simulink model "Dynamic_obstacle_avoidance_PIL"  (R2019a)
settings: Solver=VariableStepAuto  StartTime=0.0  StopTime=distance/V  MaxStep=1e-3  RelTol=1e-3  EnableMultiTasking=on
undefined symbols (not defined in the file): extended_map, fakeObs, Lw, obstacle, p, param, Ts, u0, WMV, WMVR, WOV, x0_dyn
libraries: simulink x4, mpclib x2
settings Model: Creator=The MathWorks, Inc.  LastModifiedBy=djtn
settings SolverCC: AlgebraicLoopSolver=LineSearch  MinimalZcImpactIntegration=on
settings DataIOCC: LimitDataPoints=on  SaveFormat=Array  SaveOutput=off  DSMLogging=off  SaveTime=off  ReturnWorkspaceOutputs=off
settings OptimizationCC: DefaultParameterBehavior=Inlined  UseDivisionForNetSlopeComputation=on  EnhancedBackFolding=on  PassReuseOutputArgsAs=Individual arguments  OptimizeBlockOrder=speed  DifferentSizesBufferReuse=on  OptimizationCustomize=off
settings DebuggingCC: AlgebraicLoopMsg=none  UnderspecifiedInitializationDetection=Classic  MergeDetectMultiDrivingBlocksExec=none  SolverPrmCheckMsg=warning  ParameterTunabilityLossMsg=error  AllowSymbolicDim=off  StateNameClashWarn=warning  SFUnexpectedBacktrackingDiag=warning  SFNoUnconditionalDefaultTransitionDiag=warning  SFExecutionAtInitializationDiag=none  UnderSpecifiedDimensionMsg=warning  ArithmeticOperatorsInVariantConditions=warning
settings HardwareCC: ProdBitPerPointer=32  ProdBitPerSizeT=32  ProdBitPerPtrDiffT=32  ProdLargestAtomicInteger=Long  ProdWordSize=32  ProdHWDeviceType=STM32CortexM
settings ModelReferenceCC: PropagateSignalLabelsOutOfModel=off
settings SFSimCC: SimUseLocalCustomCode=off  MATLABDynamicMemAlloc=off
settings RTWCC: SystemTargetFile=stm32.tlc  TemplateMakefile=stm32.tmf  Description=stm32 (Embedded Target)  GenerateReport=on  RTWUseLocalCustomCode=off  IncludeHyperlinkInReport=on  GenerateTraceInfo=on  GenerateTraceReport=on  GenerateTraceReportSl=on  GenerateTraceReportSf=on  GenerateTraceReportEml=on  CheckMdlBeforeBuild=Warning
settings CodeAppCC: ForceParamTrailComments=on  IgnoreCustomStorageClasses=off  MaxIdLength=64  OperatorAnnotations=on  SimulinkDataObjDesc=on  SFDataObjDesc=on  CustomSymbolStrType=$N$R$M  SimulinkBlockComments=off
settings STFCustomTargetCC: CodeReplacementLibrary=ARM CMSIS SIN COS  MultiwordLength=256  ParMdlRefBuildCompliant=on  IncludeMdlTerminateFcn=off  CombineOutputUpdateFcns=on  ERTCustomFileBanners=on  SupportContinuousTime=off  SupportNonInlinedSFcns=off  RemoveResetFunc=on  MATLABClassNameForMDSCustomization=Simulink.SoftwareTarget.ERTCustomization  GRTInterface=off  SystemTargetFile=stm32.tlc
settings ERTTargetCC: CodeReplacementLibrary=ARM CMSIS SIN COS  CompOptLevelCompliant=off  ConcurrentExecutionCompliant=off  IncludeMdlTerminateFcn=off  ModelStepFunctionPrototypeControlCompliant=off  CPPClassGenCompliant=off  UseToolchainInfoCompliant=off  ExtModeStaticAllocSize=256  ExtModeMexFile=ext_serial_win32_comm  ExtModeMexArgs=0,1,115200,10  InlinedParameterPlacement=NonHierarchical  ERTSrcFileBannerTemplate=sourceFileTemplate.cgt  ERTHdrFileBannerTemplate=sourceFileTemplate.cgt  ERTDataSrcFileTemplate=sourceFileTemplate.cgt  ERTDataHdrFileTemplate=sourceFileTemplate.cgt  ERTCustomFileTemplate=customRoutineProcess.tlc
settings ConfigComp: CovMetricSettings=dw  CovSaveCumulativeToWorkspaceVar=on  CovSaveSingleToWorkspaceVar=on  CovExternalEMLEnable=off  CovSFcnEnable=off
settings SimscapeCC: SimscapeNormalizeSystem=off  SimscapeNominalValues="[{\"value\":\"10\",\"unit\":\"V\"},{\"value\":\"1\",\"unit\":\"A\"},{\"value\":\"10\",\"unit\":\"N*m\"},{\"value\":\"10\",\"unit\":\"bar\"},{\"value\":\"100\",\"unit\":\"kJ/kg\"},{\"value\":\"1\",\"unit\":\"kW\"},{\"value\":\"300\",\"unit\":\"K\"},{\"value\":\"100\",\"unit\":\"cm^3/s\"},{\"value\":\"1\",\"unit\":\"kN\"},{\"value\":\"1\",\"unit\":\"g/cm^3\"},{\"value\":\"1\",\"unit\":\"l\"},{\"value\":\"1\",\"unit\":\"cm^2\"},{\"value\":\"60\",\"unit\":\"Hz\"}]"
settings ConfigurationSet: Description=SimMechanics 2G
settings ExplorerConfigSet: InternalSimMechanicsExplorerSettings="<ExplorerConfiguration><canonicalview>default</canonicalview><AnimationSetting><BasePlaybackSpeed>1.0</BasePlaybackSpeed><PlaybackSpeedFactor>1.0</PlaybackSpeedFactor></AnimationSetting><TilePanel><TileInfo><Tiles Columns=\"1\" Count=\"1\" Rows=\"1\"><Column Left=\"2\" Weight=\"1\"/><Column Left=\"1552\"/><Row Top=\"2\" Weight=\"1\"/><Row Top=\"932\"/><Tile Height=\"1\" Width=\"1\" X=\"0\" Y=\"0\"/></Tiles></TileInfo><SceneInfo><SceneViewer><BGColor><R>0.60000002384185791</R><G>0.60000002384185791</G><B>0.60000002384185791</B></BGColor><Camera><Position><X>0.027865189060748197</X><Y>-2.5719092456962986</Y><Z>0.23157896538506753</Z></Position><Center><X>0.62659712312732463</X><Y>-0.46110119691712204</Y><Z>0.22087365386473376</Z></Center><Up><X>-0.0079438354874226333</X><Y>0.0073246425924307582</Y><Z>0.99994162084025784</Z></Up><Left>-0.24533778208815546</Left><Right>0.24533778208815546</Right><Bottom>-0.79734779727023208</Bottom><Top>0.79734779727023208</Top></Camera></SceneViewer></SceneInfo></TilePanel></ExplorerConfiguration>"

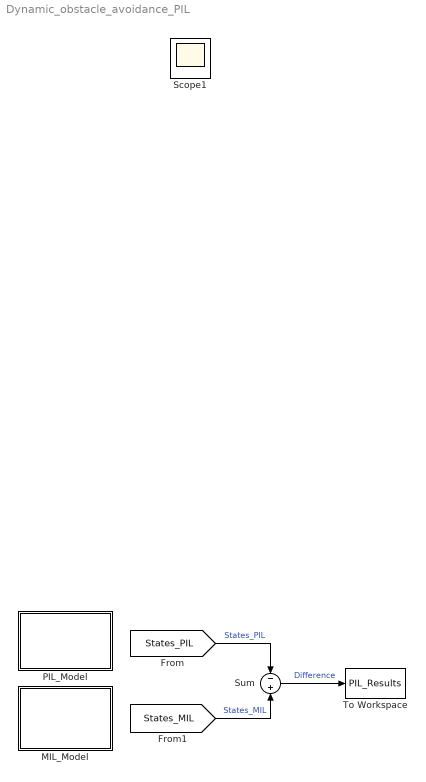
== system Dynamic_obstacle_avoidance_PIL ==
  MIL_Model : Subsystem
  PIL_Model : Subsystem
  Sum : Sum  Inputs=-+
  To Workspace : ToWorkspace  VariableName=PIL_Results  SampleTime=Ts
  Scope1 : Scope
  wires:
  [States_PIL] -> Sum/1  "States_PIL"
  [States_MIL] -> Sum/2  "States_MIL"
  Sum/1 -> To Workspace/1  "Difference"

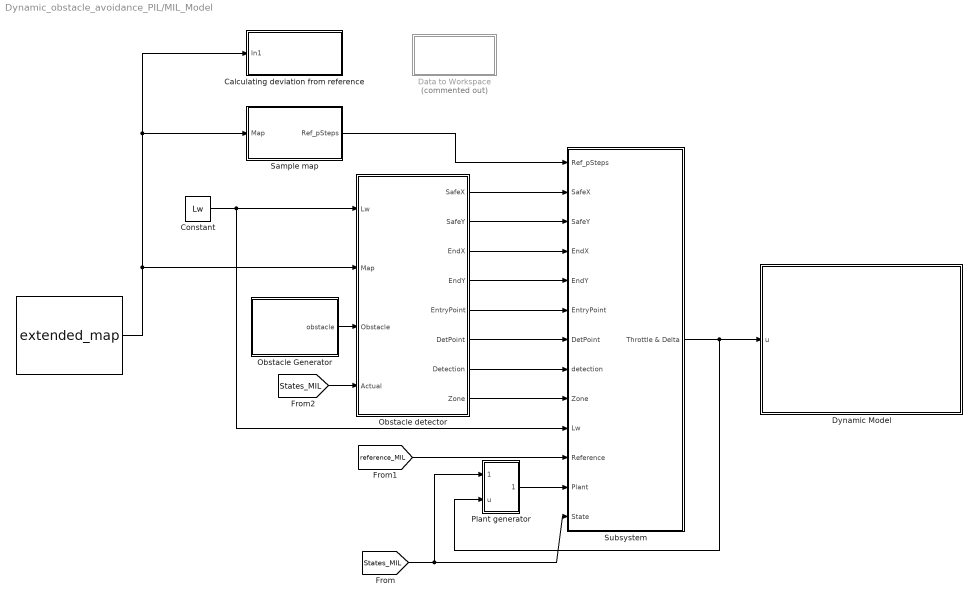
== system Dynamic_obstacle_avoidance_PIL/MIL_Model ==
  "  " : Constant  Value=extended_map  SampleTime=Ts
      mask Display: image('creative_map_city.jpg')
  Calculating deviation from reference : Subsystem
  Constant : Constant  Value=Lw
  Data to Workspace : Subsystem  Commented=on
  Dynamic Model : Subsystem
      mask Display: image('hyundai_verna.jpg')
  Obstacle Generator : Subsystem
  Obstacle detector : Subsystem
  Plant generator : Subsystem
  Sample map : Subsystem
  Subsystem : Subsystem
  wires:
  Obstacle detector/8(Zone) -> Subsystem/9(Zone)
  Obstacle detector/7(Detection) -> Subsystem/8(detection)
  Obstacle detector/6(DetPoint) -> Subsystem/7(DetPoint)
  Obstacle detector/5(EntryPoint) -> Subsystem/6(EntryPoint)
  Obstacle detector/4(EndY) -> Subsystem/5(EndY)
  Obstacle detector/3(EndX) -> Subsystem/4(EndX)
  Obstacle detector/2(SafeY) -> Subsystem/3(SafeY)
  Obstacle detector/1(SafeX) -> Subsystem/2(SafeX)
  [States_MIL] -> Obstacle detector/4(Actual)
  Obstacle Generator/1(obstacle) -> Obstacle detector/3(Obstacle)
  Sample map/1(Ref_pSteps) -> Subsystem/1(Ref_pSteps)
  "  "/1 -> Obstacle detector/2(Map), Sample map/1(Map), Calculating deviation from reference/1(In1)
  Plant generator/1(Out1) -> Subsystem/12(Plant)
  [reference_MIL] -> Subsystem/11(Reference)
  Subsystem/1(Throttle & Delta) -> Plant generator/2(u), Dynamic Model/1(u)
  Constant/1 -> Subsystem/10("Lw "), Obstacle detector/1(Lw)
  [States_MIL] -> Subsystem/13(State), Plant generator/1(State)

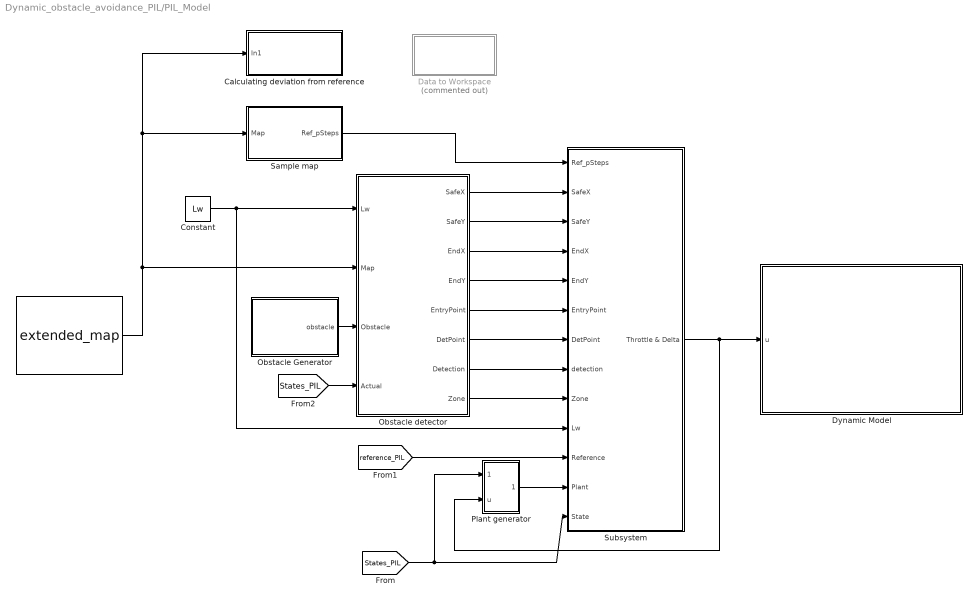
== system Dynamic_obstacle_avoidance_PIL/PIL_Model ==
  "  " : Constant  Value=extended_map  SampleTime=Ts
      mask Display: image('creative_map_city.jpg')
  Calculating deviation from reference : Subsystem
  Constant : Constant  Value=Lw
  Data to Workspace : Subsystem  Commented=on
  Dynamic Model : Subsystem
      mask Display: image('hyundai_verna.jpg')
  Obstacle Generator : Subsystem
  Obstacle detector : Subsystem
  Plant generator : Subsystem
  Sample map : Subsystem
  Subsystem : Subsystem
  wires:
  [States_PIL] -> Plant generator/1(State), Subsystem/13(State)
  Constant/1 -> Obstacle detector/1(Lw), Subsystem/10("Lw ")
  Subsystem/1(Throttle & Delta) -> Dynamic Model/1(u), Plant generator/2(u)
  [reference_PIL] -> Subsystem/11(Reference)
  Plant generator/1(Out1) -> Subsystem/12(Plant)
  "  "/1 -> Calculating deviation from reference/1(In1), Sample map/1(Map), Obstacle detector/2(Map)
  Sample map/1(Ref_pSteps) -> Subsystem/1(Ref_pSteps)
  Obstacle Generator/1(obstacle) -> Obstacle detector/3(Obstacle)
  [States_PIL] -> Obstacle detector/4(Actual)
  Obstacle detector/1(SafeX) -> Subsystem/2(SafeX)
  Obstacle detector/2(SafeY) -> Subsystem/3(SafeY)
  Obstacle detector/3(EndX) -> Subsystem/4(EndX)
  Obstacle detector/4(EndY) -> Subsystem/5(EndY)
  Obstacle detector/5(EntryPoint) -> Subsystem/6(EntryPoint)
  Obstacle detector/6(DetPoint) -> Subsystem/7(DetPoint)
  Obstacle detector/7(Detection) -> Subsystem/8(detection)
  Obstacle detector/8(Zone) -> Subsystem/9(Zone)

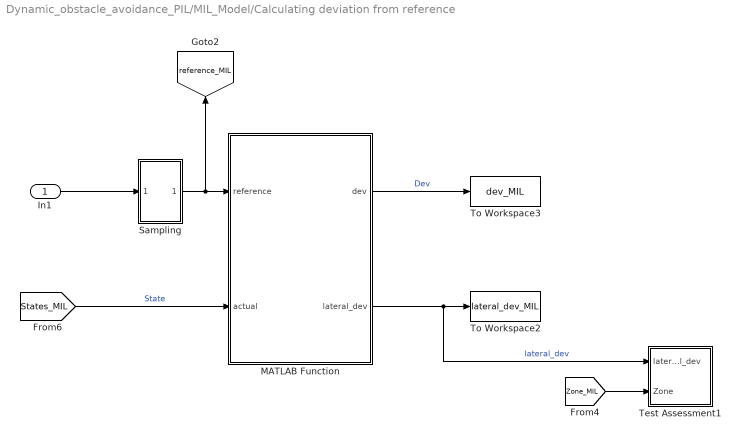
== system Dynamic_obstacle_avoidance_PIL/MIL_Model/Calculating deviation from reference ==
  In1 : Inport
  MATLAB Function : MATLAB Function  TreatAsAtomicUnit=on
  Sampling : Subsystem
  Test Assessment1 : Test Sequence  TreatAsAtomicUnit=on
  To Workspace2 : ToWorkspace  VariableName=lateral_dev_MIL  SampleTime=Ts
  To Workspace3 : ToWorkspace  VariableName=dev_MIL  SampleTime=-1
  tag scope: reference_MIL=global
  wires:
  [Zone_MIL] -> Test Assessment1/2(Zone)
  MATLAB Function/2(lateral_dev) -> Test Assessment1/1(lateral_dev), To Workspace2/1  "lateral_dev"
  MATLAB Function/1(dev) -> To Workspace3/1  "Dev"
  In1/1 -> Sampling/1(In1)
  Sampling/1(Out1) -> [reference_MIL], MATLAB Function/1(reference)
  [States_MIL] -> MATLAB Function/2(actual)  "State"

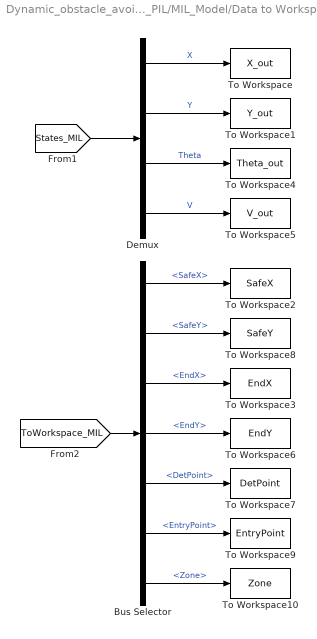
== system Dynamic_obstacle_avoidance_PIL/MIL_Model/Data to Workspace ==
  Bus Selector : BusSelector  OutputSignals=SafeX,SafeY,EndX,EndY,DetPoint,EntryPoint,Zone
  Demux : Demux
  To Workspace : ToWorkspace  VariableName=X_out  SampleTime=Ts
  To Workspace1 : ToWorkspace  VariableName=Y_out  SampleTime=Ts
  To Workspace10 : ToWorkspace  VariableName=Zone  SampleTime=-1
  To Workspace2 : ToWorkspace  VariableName=SafeX  SampleTime=-1
  To Workspace3 : ToWorkspace  VariableName=EndX  SampleTime=-1
  To Workspace4 : ToWorkspace  VariableName=Theta_out  SampleTime=Ts
  To Workspace5 : ToWorkspace  VariableName=V_out  SampleTime=Ts
  To Workspace6 : ToWorkspace  VariableName=EndY  SampleTime=-1
  To Workspace7 : ToWorkspace  VariableName=DetPoint  SampleTime=-1
  To Workspace8 : ToWorkspace  VariableName=SafeY  SampleTime=-1
  To Workspace9 : ToWorkspace  VariableName=EntryPoint  SampleTime=-1
  wires:
  Bus Selector/7 -> To Workspace10/1  "<Zone>"
  Bus Selector/6 -> To Workspace9/1  "<EntryPoint>"
  Bus Selector/5 -> To Workspace7/1  "<DetPoint>"
  Bus Selector/4 -> To Workspace6/1  "<EndY>"
  Bus Selector/3 -> To Workspace3/1  "<EndX>"
  Bus Selector/2 -> To Workspace8/1  "<SafeY>"
  Bus Selector/1 -> To Workspace2/1  "<SafeX>"
  [ToWorkspace_MIL] -> Bus Selector/1
  Demux/1 -> To Workspace/1  "X"
  [States_MIL] -> Demux/1
  Demux/4 -> To Workspace5/1  "V"
  Demux/2 -> To Workspace1/1  "Y"
  Demux/3 -> To Workspace4/1  "Theta"

== system Dynamic_obstacle_avoidance_PIL/MIL_Model/Dynamic Model ==
  u : Inport
  Bus Creator1 : BusCreator  Inputs=4
  C_r : Constant  Value=param  SampleTime=Ts
  Dynamic_Model : MATLAB Function  TreatAsAtomicUnit=on
  Integrator : Integrator  InitialCondition=x0_dyn
  Lateral Acceleration Assessment : Test Sequence  TreatAsAtomicUnit=on
  Selector2 : Selector  InputPortWidth=6  IndexOptions=Index vector (dialog)  Indices=[5]  OutputSizes=1
  tag scope: States_MIL=global
  wires:
  u/1 -> Dynamic_Model/2(u)
  C_r/1 -> Dynamic_Model/3(param)
  Integrator/1 -> Dynamic_Model/1(x)
  Dynamic_Model/5(v) -> Bus Creator1/4  "V"
  Dynamic_Model/2(X) -> Bus Creator1/1  "X"
  Dynamic_Model/4(yaw) -> Bus Creator1/3  "yaw"
  Dynamic_Model/1(xdot) -> Selector2/1, Integrator/1
  Selector2/1 -> Lateral Acceleration Assessment/1(Lateral_acceleration)  "Lateral acceleration"
  Bus Creator1/1 -> [States_MIL]
  Dynamic_Model/3(Y) -> Bus Creator1/2  "Y"

== system Dynamic_obstacle_avoidance_PIL/MIL_Model/Obstacle Generator ==
  Constant4 : Constant  Value=obstacle
  FakeObs : Constant  Value=fakeObs
  From Workspace : FromWorkspace  VariableName=extended_obs  SampleTime=0
  From Workspace1 : FromWorkspace  VariableName=extended_obs2  SampleTime=0
  Matrix Concatenate : Concatenate  NumInputs=4  Mode=Multidimensional array
  Transpose : Math  Operator=transpose  SaturateOnIntegerOverflow=on
  Transpose1 : Math  Operator=transpose  SaturateOnIntegerOverflow=on
  obstacle : Outport
  wires:
  FakeObs/1 -> Matrix Concatenate/4
  Transpose1/1 -> Matrix Concatenate/3
  From Workspace1/1 -> Transpose1/1
  Transpose/1 -> Matrix Concatenate/2
  Constant4/1 -> Matrix Concatenate/1
  Matrix Concatenate/1 -> obstacle/1
  From Workspace/1 -> Transpose/1

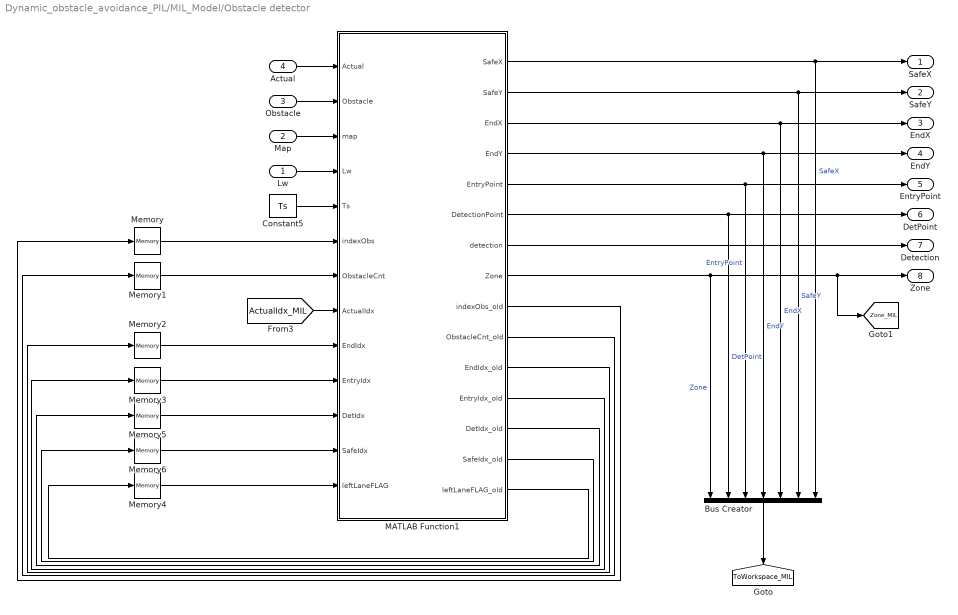
== system Dynamic_obstacle_avoidance_PIL/MIL_Model/Obstacle detector ==
  Lw : Inport
  Map : Inport  Port=2
  Obstacle : Inport  Port=3
  Actual : Inport  Port=4
  Bus Creator : BusCreator  Inputs=7
  Constant5 : Constant  Value=Ts
  MATLAB Function1 : MATLAB Function  TreatAsAtomicUnit=on
  Memory{,1..6} (7 alike) : Memory
  SafeX : Outport
  SafeY : Outport  Port=2
  EndX : Outport  Port=3
  EndY : Outport  Port=4
  EntryPoint : Outport  Port=5
  DetPoint : Outport  Port=6
  Detection : Outport  Port=7
  Zone : Outport  Port=8
  tag scope: ToWorkspace_MIL=global, Zone_MIL=global
  wires:
  Map/1 -> MATLAB Function1/3(map)
  MATLAB Function1/12(EntryIdx_old) -> Memory3/1
  MATLAB Function1/13(DetIdx_old) -> Memory5/1
  MATLAB Function1/14(SafeIdx_old) -> Memory6/1
  Constant5/1 -> MATLAB Function1/5(Ts)
  Memory/1 -> MATLAB Function1/6(indexObs)
  MATLAB Function1/9(indexObs_old) -> Memory/1
  MATLAB Function1/4(EndY) -> Bus Creator/4, EndY/1  "EndY"
  MATLAB Function1/3(EndX) -> Bus Creator/5, EndX/1  "EndX"
  Obstacle/1 -> MATLAB Function1/2(Obstacle)
  Memory5/1 -> MATLAB Function1/11(DetIdx)
  MATLAB Function1/7(detection) -> Detection/1
  Memory2/1 -> MATLAB Function1/9(EndIdx)
  Memory6/1 -> MATLAB Function1/12(SafeIdx)
  Memory4/1 -> MATLAB Function1/13(leftLaneFLAG)
  Memory1/1 -> MATLAB Function1/7(ObstacleCnt)
  MATLAB Function1/5(EntryPoint) -> EntryPoint/1, Bus Creator/3  "EntryPoint"
  Bus Creator/1 -> [ToWorkspace_MIL]
  MATLAB Function1/2(SafeY) -> Bus Creator/6, SafeY/1  "SafeY"
  Actual/1 -> MATLAB Function1/1(Actual)
  MATLAB Function1/1(SafeX) -> Bus Creator/7, SafeX/1  "SafeX"
  MATLAB Function1/15(leftLaneFLAG_old) -> Memory4/1
  MATLAB Function1/6(DetectionPoint) -> DetPoint/1, Bus Creator/2  "DetPoint"
  MATLAB Function1/10(ObstacleCnt_old) -> Memory1/1
  MATLAB Function1/11(EndIdx_old) -> Memory2/1
  MATLAB Function1/8(Zone) -> Bus Creator/1, [Zone_MIL], Zone/1  "Zone"
  Memory3/1 -> MATLAB Function1/10(EntryIdx)
  [ActualIdx_MIL] -> MATLAB Function1/8(ActualIdx)
  Lw/1 -> MATLAB Function1/4(Lw)

== system Dynamic_obstacle_avoidance_PIL/MIL_Model/Plant generator ==
  State : Inport
  u : Inport  Port=2
  " " : Constant  Value=param(1:2)  SampleTime=Ts
  Bus Creator2 : BusCreator  Inputs=8
  Plant Model Generator : MATLAB Function  TreatAsAtomicUnit=on
  Out1 : Outport  VectorParamsAs1DForOutWhenUnconnected=on
  wires:
  State/1 -> Plant Model Generator/1(x)
  Bus Creator2/1 -> Out1/1
  Plant Model Generator/8(DX) -> Bus Creator2/8
  Plant Model Generator/1(A) -> Bus Creator2/1
  Plant Model Generator/4(D) -> Bus Creator2/4
  Plant Model Generator/5(U) -> Bus Creator2/5
  u/1 -> Plant Model Generator/2(u)
  Plant Model Generator/7(X) -> Bus Creator2/7
  Plant Model Generator/2(B) -> Bus Creator2/2
  Plant Model Generator/3(C) -> Bus Creator2/3
  Plant Model Generator/6(Y) -> Bus Creator2/6
  " "/1 -> Plant Model Generator/3(param)

== system Dynamic_obstacle_avoidance_PIL/MIL_Model/Sample map ==
  Map : Inport
  Constant1 : Constant  Value=2
  Counter Free-Running : simulink/Sources/Counter Free-Running  NumBits=32  tsamp=Ts
  Selector : Selector  NumberOfDimensions=2  InputPortWidth=3  IndexOptions=Starting index (port),Select all  Indices=[1 3],1  OutputSizes=p,1
  Sum : Sum  Inputs=|++
  Ref_pSteps : Outport
  wires:
  Map/1 -> Selector/1
  Counter Free-Running/1 -> Sum/1
  Selector/1 -> Ref_pSteps/1
  Constant1/1 -> Sum/2
  Sum/1 -> Selector/2

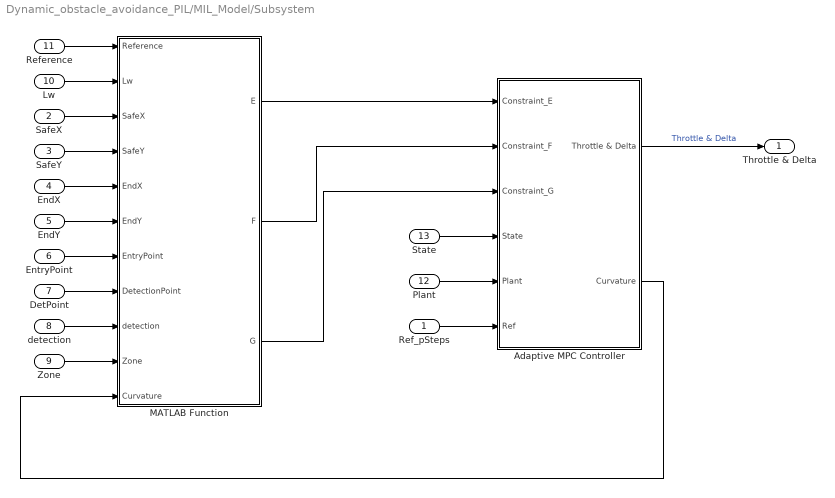
== system Dynamic_obstacle_avoidance_PIL/MIL_Model/Subsystem ==
  Ref_pSteps : Inport
  SafeX : Inport  Port=2
  SafeY : Inport  Port=3
  EndX : Inport  Port=4
  EndY : Inport  Port=5
  EntryPoint : Inport  Port=6
  DetPoint : Inport  Port=7
  detection : Inport  Port=8
  Zone : Inport  Port=9
  "Lw " : Inport  Port=10
  Reference : Inport  Port=11
  Plant : Inport  Port=12
  State : Inport  Port=13
  Adaptive MPC Controller : Subsystem
  MATLAB Function : MATLAB Function  TreatAsAtomicUnit=on
  Throttle & Delta : Outport
  wires:
  Ref_pSteps/1 -> Adaptive MPC Controller/6(Ref)
  Adaptive MPC Controller/2(Curvature) -> MATLAB Function/11(Curvature)
  Adaptive MPC Controller/1(Throttle & Delta) -> Throttle & Delta/1  "Throttle & Delta"
  MATLAB Function/2(F) -> Adaptive MPC Controller/2(Constraint_F)
  MATLAB Function/3(G) -> Adaptive MPC Controller/3(Constraint_G)
  MATLAB Function/1(E) -> Adaptive MPC Controller/1(Constraint_E)
  State/1 -> Adaptive MPC Controller/4(State)
  Plant/1 -> Adaptive MPC Controller/5(Plant)
  Zone/1 -> MATLAB Function/10(Zone)
  detection/1 -> MATLAB Function/9(detection)
  DetPoint/1 -> MATLAB Function/8(DetectionPoint)
  EntryPoint/1 -> MATLAB Function/7(EntryPoint)
  EndY/1 -> MATLAB Function/6(EndY)
  EndX/1 -> MATLAB Function/5(EndX)
  SafeY/1 -> MATLAB Function/4(SafeY)
  SafeX/1 -> MATLAB Function/3(SafeX)
  "Lw "/1 -> MATLAB Function/2(Lw)
  Reference/1 -> MATLAB Function/1(Reference)

== system Dynamic_obstacle_avoidance_PIL/PIL_Model/Calculating deviation from reference ==
  In1 : Inport
  MATLAB Function : MATLAB Function  TreatAsAtomicUnit=on
  Sampling : Subsystem
  Test Assessment1 : Test Sequence  TreatAsAtomicUnit=on
  To Workspace2 : ToWorkspace  VariableName=lateral_dev_PIL  SampleTime=Ts
  To Workspace3 : ToWorkspace  VariableName=dev_PIL  SampleTime=-1
  tag scope: reference_PIL=global
  wires:
  [States_PIL] -> MATLAB Function/2(actual)  "State"
  Sampling/1(Out1) -> MATLAB Function/1(reference), [reference_PIL]
  In1/1 -> Sampling/1(In1)
  MATLAB Function/1(dev) -> To Workspace3/1  "Dev"
  MATLAB Function/2(lateral_dev) -> To Workspace2/1, Test Assessment1/1(lateral_dev)  "lateral_dev"
  [Zone_PIL] -> Test Assessment1/2(Zone)

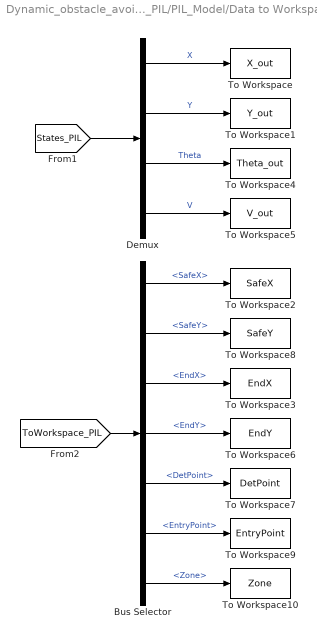
== system Dynamic_obstacle_avoidance_PIL/PIL_Model/Data to Workspace ==
  Bus Selector : BusSelector  OutputSignals=SafeX,SafeY,EndX,EndY,DetPoint,EntryPoint,Zone
  Demux : Demux
  To Workspace : ToWorkspace  VariableName=X_out  SampleTime=Ts
  To Workspace1 : ToWorkspace  VariableName=Y_out  SampleTime=Ts
  To Workspace10 : ToWorkspace  VariableName=Zone  SampleTime=-1
  To Workspace2 : ToWorkspace  VariableName=SafeX  SampleTime=-1
  To Workspace3 : ToWorkspace  VariableName=EndX  SampleTime=-1
  To Workspace4 : ToWorkspace  VariableName=Theta_out  SampleTime=Ts
  To Workspace5 : ToWorkspace  VariableName=V_out  SampleTime=Ts
  To Workspace6 : ToWorkspace  VariableName=EndY  SampleTime=-1
  To Workspace7 : ToWorkspace  VariableName=DetPoint  SampleTime=-1
  To Workspace8 : ToWorkspace  VariableName=SafeY  SampleTime=-1
  To Workspace9 : ToWorkspace  VariableName=EntryPoint  SampleTime=-1
  wires:
  Demux/3 -> To Workspace4/1  "Theta"
  Demux/2 -> To Workspace1/1  "Y"
  Demux/4 -> To Workspace5/1  "V"
  [States_PIL] -> Demux/1
  Demux/1 -> To Workspace/1  "X"
  [ToWorkspace_PIL] -> Bus Selector/1
  Bus Selector/1 -> To Workspace2/1  "<SafeX>"
  Bus Selector/2 -> To Workspace8/1  "<SafeY>"
  Bus Selector/3 -> To Workspace3/1  "<EndX>"
  Bus Selector/4 -> To Workspace6/1  "<EndY>"
  Bus Selector/5 -> To Workspace7/1  "<DetPoint>"
  Bus Selector/6 -> To Workspace9/1  "<EntryPoint>"
  Bus Selector/7 -> To Workspace10/1  "<Zone>"

== system Dynamic_obstacle_avoidance_PIL/PIL_Model/Dynamic Model ==
  u : Inport
  Bus Creator1 : BusCreator  Inputs=4
  C_r : Constant  Value=param  SampleTime=Ts
  Dynamic_Model : MATLAB Function  TreatAsAtomicUnit=on
  Integrator : Integrator  InitialCondition=x0_dyn
  Lateral Acceleration Assessment : Test Sequence  TreatAsAtomicUnit=on
  Selector2 : Selector  InputPortWidth=6  IndexOptions=Index vector (dialog)  Indices=[5]  OutputSizes=1
  tag scope: States_PIL=global
  wires:
  Dynamic_Model/3(Y) -> Bus Creator1/2  "Y"
  Bus Creator1/1 -> [States_PIL]
  Selector2/1 -> Lateral Acceleration Assessment/1(Lateral_acceleration)  "Lateral acceleration"
  Dynamic_Model/1(xdot) -> Integrator/1, Selector2/1
  Dynamic_Model/4(yaw) -> Bus Creator1/3  "yaw"
  Dynamic_Model/2(X) -> Bus Creator1/1  "X"
  Dynamic_Model/5(v) -> Bus Creator1/4  "V"
  Integrator/1 -> Dynamic_Model/1(x)
  C_r/1 -> Dynamic_Model/3(param)
  u/1 -> Dynamic_Model/2(u)

== system Dynamic_obstacle_avoidance_PIL/PIL_Model/Obstacle Generator ==
  Constant4 : Constant  Value=obstacle
  FakeObs : Constant  Value=fakeObs
  From Workspace : FromWorkspace  VariableName=extended_obs  SampleTime=0
  From Workspace1 : FromWorkspace  VariableName=extended_obs2  SampleTime=0
  Matrix Concatenate : Concatenate  NumInputs=4  Mode=Multidimensional array
  Transpose : Math  Operator=transpose  SaturateOnIntegerOverflow=on
  Transpose1 : Math  Operator=transpose  SaturateOnIntegerOverflow=on
  obstacle : Outport
  wires:
  From Workspace/1 -> Transpose/1
  Matrix Concatenate/1 -> obstacle/1
  Constant4/1 -> Matrix Concatenate/1
  Transpose/1 -> Matrix Concatenate/2
  From Workspace1/1 -> Transpose1/1
  Transpose1/1 -> Matrix Concatenate/3
  FakeObs/1 -> Matrix Concatenate/4

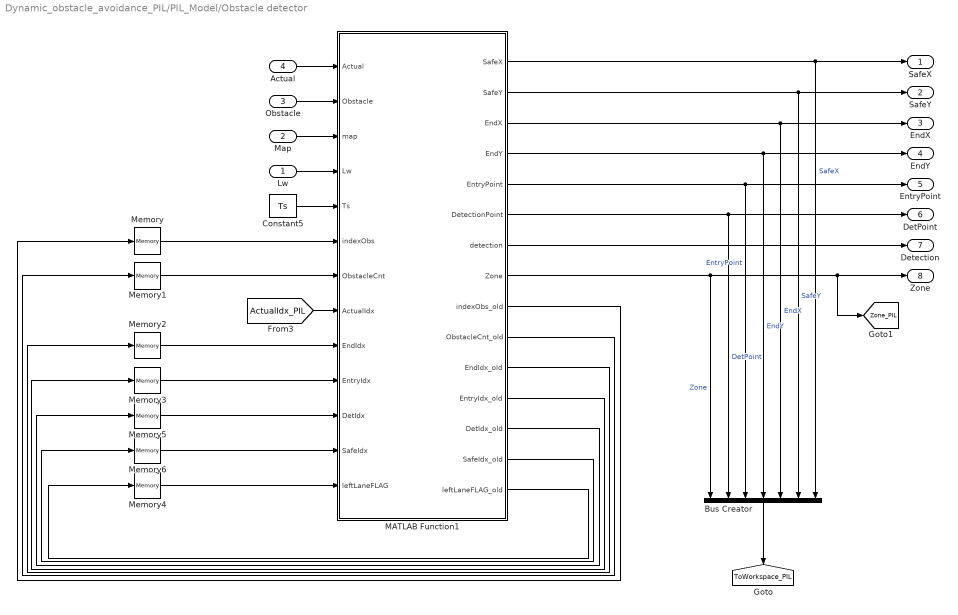
== system Dynamic_obstacle_avoidance_PIL/PIL_Model/Obstacle detector ==
  Lw : Inport
  Map : Inport  Port=2
  Obstacle : Inport  Port=3
  Actual : Inport  Port=4
  Bus Creator : BusCreator  Inputs=7
  Constant5 : Constant  Value=Ts
  MATLAB Function1 : MATLAB Function  TreatAsAtomicUnit=on
  Memory{,1..6} (7 alike) : Memory
  SafeX : Outport
  SafeY : Outport  Port=2
  EndX : Outport  Port=3
  EndY : Outport  Port=4
  EntryPoint : Outport  Port=5
  DetPoint : Outport  Port=6
  Detection : Outport  Port=7
  Zone : Outport  Port=8
  tag scope: ToWorkspace_PIL=global, Zone_PIL=global
  wires:
  Lw/1 -> MATLAB Function1/4(Lw)
  [ActualIdx_PIL] -> MATLAB Function1/8(ActualIdx)
  Memory3/1 -> MATLAB Function1/10(EntryIdx)
  MATLAB Function1/8(Zone) -> Zone/1, [Zone_PIL], Bus Creator/1  "Zone"
  MATLAB Function1/11(EndIdx_old) -> Memory2/1
  MATLAB Function1/10(ObstacleCnt_old) -> Memory1/1
  MATLAB Function1/6(DetectionPoint) -> Bus Creator/2, DetPoint/1  "DetPoint"
  MATLAB Function1/15(leftLaneFLAG_old) -> Memory4/1
  MATLAB Function1/1(SafeX) -> SafeX/1, Bus Creator/7  "SafeX"
  Actual/1 -> MATLAB Function1/1(Actual)
  MATLAB Function1/2(SafeY) -> SafeY/1, Bus Creator/6  "SafeY"
  Bus Creator/1 -> [ToWorkspace_PIL]
  MATLAB Function1/5(EntryPoint) -> Bus Creator/3, EntryPoint/1  "EntryPoint"
  Memory1/1 -> MATLAB Function1/7(ObstacleCnt)
  Memory4/1 -> MATLAB Function1/13(leftLaneFLAG)
  Memory6/1 -> MATLAB Function1/12(SafeIdx)
  Memory2/1 -> MATLAB Function1/9(EndIdx)
  MATLAB Function1/7(detection) -> Detection/1
  Memory5/1 -> MATLAB Function1/11(DetIdx)
  Obstacle/1 -> MATLAB Function1/2(Obstacle)
  MATLAB Function1/3(EndX) -> EndX/1, Bus Creator/5  "EndX"
  MATLAB Function1/4(EndY) -> EndY/1, Bus Creator/4  "EndY"
  MATLAB Function1/9(indexObs_old) -> Memory/1
  Memory/1 -> MATLAB Function1/6(indexObs)
  Constant5/1 -> MATLAB Function1/5(Ts)
  MATLAB Function1/14(SafeIdx_old) -> Memory6/1
  MATLAB Function1/13(DetIdx_old) -> Memory5/1
  MATLAB Function1/12(EntryIdx_old) -> Memory3/1
  Map/1 -> MATLAB Function1/3(map)

== system Dynamic_obstacle_avoidance_PIL/PIL_Model/Plant generator ==
  State : Inport
  u : Inport  Port=2
  " " : Constant  Value=param(1:2)  SampleTime=Ts
  Bus Creator2 : BusCreator  Inputs=8
  Plant Model Generator : MATLAB Function  TreatAsAtomicUnit=on
  Out1 : Outport  VectorParamsAs1DForOutWhenUnconnected=on
  wires:
  " "/1 -> Plant Model Generator/3(param)
  Plant Model Generator/6(Y) -> Bus Creator2/6
  Plant Model Generator/3(C) -> Bus Creator2/3
  Plant Model Generator/2(B) -> Bus Creator2/2
  Plant Model Generator/7(X) -> Bus Creator2/7
  u/1 -> Plant Model Generator/2(u)
  Plant Model Generator/5(U) -> Bus Creator2/5
  Plant Model Generator/4(D) -> Bus Creator2/4
  Plant Model Generator/1(A) -> Bus Creator2/1
  Plant Model Generator/8(DX) -> Bus Creator2/8
  Bus Creator2/1 -> Out1/1
  State/1 -> Plant Model Generator/1(x)

== system Dynamic_obstacle_avoidance_PIL/PIL_Model/Sample map ==
  Map : Inport
  Constant1 : Constant  Value=2
  Counter Free-Running : simulink/Sources/Counter Free-Running  NumBits=32  tsamp=Ts
  Selector : Selector  NumberOfDimensions=2  InputPortWidth=3  IndexOptions=Starting index (port),Select all  Indices=[1 3],1  OutputSizes=p,1
  Sum : Sum  Inputs=|++
  Ref_pSteps : Outport
  wires:
  Sum/1 -> Selector/2
  Constant1/1 -> Sum/2
  Selector/1 -> Ref_pSteps/1
  Counter Free-Running/1 -> Sum/1
  Map/1 -> Selector/1

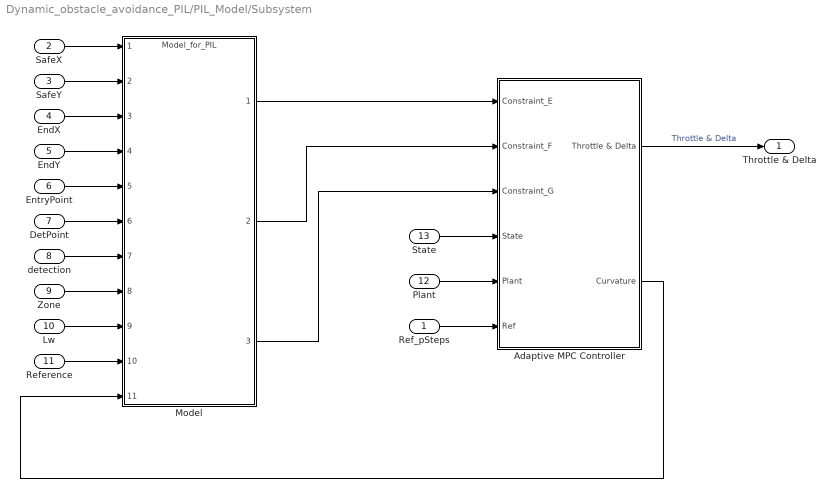
== system Dynamic_obstacle_avoidance_PIL/PIL_Model/Subsystem ==
  Ref_pSteps : Inport
  SafeX : Inport  Port=2
  SafeY : Inport  Port=3
  EndX : Inport  Port=4
  EndY : Inport  Port=5
  EntryPoint : Inport  Port=6
  DetPoint : Inport  Port=7
  detection : Inport  Port=8
  Zone : Inport  Port=9
  "Lw " : Inport  Port=10
  Reference : Inport  Port=11
  Plant : Inport  Port=12
  State : Inport  Port=13
  Adaptive MPC Controller : Subsystem
  Model : ModelReference  ModelNameDialog=Model_for_PIL.slx  SimulationMode=Processor-in-the-loop (PIL)  ModelReferenceVersion=1.18
  Throttle & Delta : Outport
  wires:
  Plant/1 -> Adaptive MPC Controller/5(Plant)
  State/1 -> Adaptive MPC Controller/4(State)
  Model/1 -> Adaptive MPC Controller/1(Constraint_E)
  Model/3 -> Adaptive MPC Controller/3(Constraint_G)
  Model/2 -> Adaptive MPC Controller/2(Constraint_F)
  Adaptive MPC Controller/1(Throttle & Delta) -> Throttle & Delta/1  "Throttle & Delta"
  Adaptive MPC Controller/2(Curvature) -> Model/11
  Ref_pSteps/1 -> Adaptive MPC Controller/6(Ref)
  SafeX/1 -> Model/1
  SafeY/1 -> Model/2
  EndX/1 -> Model/3
  EndY/1 -> Model/4
  EntryPoint/1 -> Model/5
  DetPoint/1 -> Model/6
  detection/1 -> Model/7
  Zone/1 -> Model/8
  "Lw "/1 -> Model/9
  Reference/1 -> Model/10

== system Dynamic_obstacle_avoidance_PIL/MIL_Model/Calculating deviation from reference/Sampling ==
  In1 : Inport
  Constant4 : Constant
  Counter Free-Running1 : simulink/Sources/Counter Free-Running  NumBits=32  tsamp=Ts
  Selector1 : Selector  NumberOfDimensions=2  InputPortWidth=3  IndexOptions=Starting index (port),Select all  Indices=[1 3],1  OutputSizes=1,1
  Sum1 : Sum  Inputs=|++
  Out1 : Outport  VectorParamsAs1DForOutWhenUnconnected=on
  tag scope: ActualIdx_MIL=global
  wires:
  In1/1 -> Selector1/1
  Selector1/1 -> Out1/1
  Sum1/1 -> Selector1/2, [ActualIdx_MIL]
  Constant4/1 -> Sum1/2
  Counter Free-Running1/1 -> Sum1/1

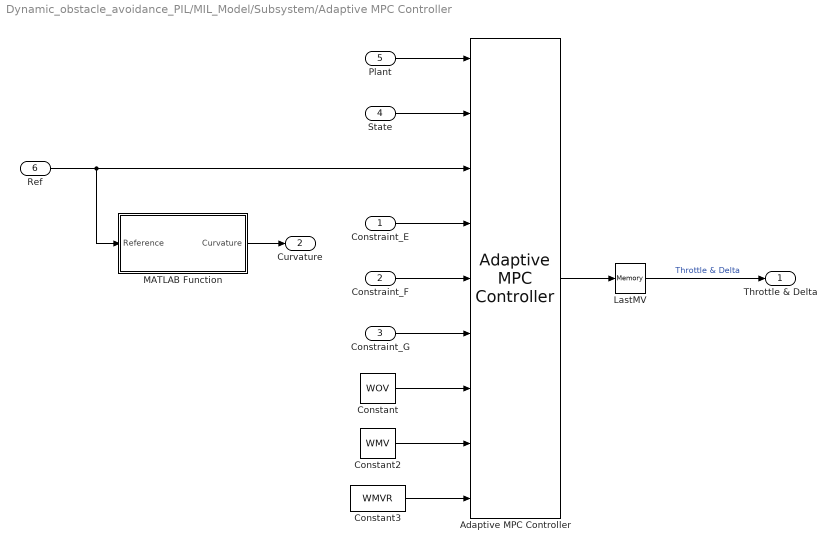
== system Dynamic_obstacle_avoidance_PIL/MIL_Model/Subsystem/Adaptive MPC Controller ==
  Constraint_E : Inport
  Constraint_F : Inport  Port=2
  Constraint_G : Inport  Port=3
  State : Inport  Port=4
  Plant : Inport  Port=5
  Ref : Inport  Port=6
  Adaptive MPC Controller : mpclib/Adaptive MPC Controller  SCDEnableBlockLinearizationSpecification=on  mpcobj=mpcobj  x0=egoStates  enable_value=0  updateMPCinCallerWorkspace=on  md_inport=off  mv_inport=off  uref_inport=off  return_cost=off  return_mvseq=off  return_qpstatus=off  return_xseq=off  return_state=off  return_ovseq=off  state_inport=off  isltv_plant=off  umin_inport=off  umax_inport=off  ymin_inport=off  ymax_inport=off  cc_inport=on  ywt_inport=on  uwt_inport=on  duwt_inport=on  rhoeps_inport=off  pm_inport=off  MaximumP=10  HorizonChoice=FixedHorizon  BlockDataType=double  SampleTimeInherited=on  switch_inport=off
  Constant : Constant  Value=WOV
  Constant2 : Constant  Value=WMV
  Constant3 : Constant  Value=WMVR
  LastMV : Memory  InitialCondition=u0
  MATLAB Function : MATLAB Function  TreatAsAtomicUnit=on
  Throttle & Delta : Outport  VectorParamsAs1DForOutWhenUnconnected=on
  Curvature : Outport  Port=2
  wires:
  Ref/1 -> MATLAB Function/1(Reference), Adaptive MPC Controller/3
  MATLAB Function/1(Curvature) -> Curvature/1
  Plant/1 -> Adaptive MPC Controller/1
  LastMV/1 -> Throttle & Delta/1  "Throttle & Delta"
  Adaptive MPC Controller/1 -> LastMV/1
  State/1 -> Adaptive MPC Controller/2
  Constant/1 -> Adaptive MPC Controller/7
  Constraint_F/1 -> Adaptive MPC Controller/5
  Constant2/1 -> Adaptive MPC Controller/8
  Constant3/1 -> Adaptive MPC Controller/9
  Constraint_G/1 -> Adaptive MPC Controller/6
  Constraint_E/1 -> Adaptive MPC Controller/4

== system Dynamic_obstacle_avoidance_PIL/PIL_Model/Calculating deviation from reference/Sampling ==
  In1 : Inport
  Constant4 : Constant
  Counter Free-Running1 : simulink/Sources/Counter Free-Running  NumBits=32  tsamp=Ts
  Selector1 : Selector  NumberOfDimensions=2  InputPortWidth=3  IndexOptions=Starting index (port),Select all  Indices=[1 3],1  OutputSizes=1,1
  Sum1 : Sum  Inputs=|++
  Out1 : Outport  VectorParamsAs1DForOutWhenUnconnected=on
  tag scope: ActualIdx_PIL=global
  wires:
  Counter Free-Running1/1 -> Sum1/1
  Constant4/1 -> Sum1/2
  Sum1/1 -> [ActualIdx_PIL], Selector1/2
  Selector1/1 -> Out1/1
  In1/1 -> Selector1/1

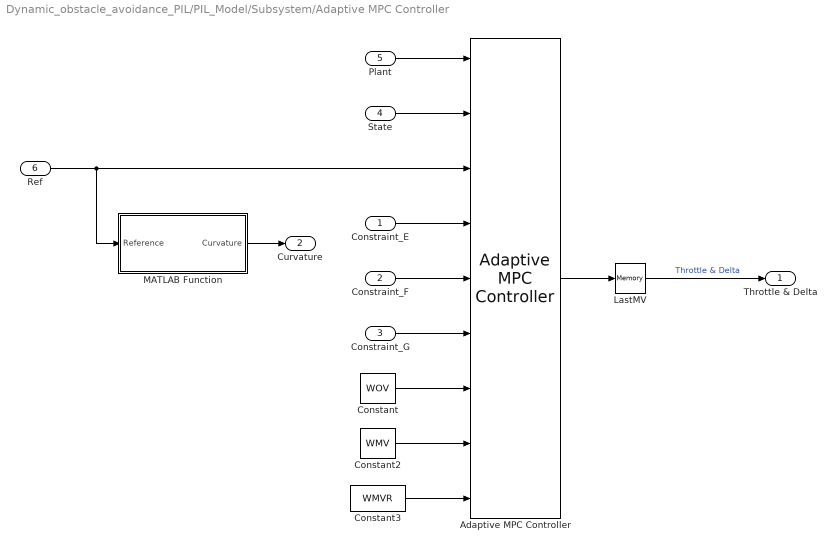
== system Dynamic_obstacle_avoidance_PIL/PIL_Model/Subsystem/Adaptive MPC Controller ==
  Constraint_E : Inport
  Constraint_F : Inport  Port=2
  Constraint_G : Inport  Port=3
  State : Inport  Port=4
  Plant : Inport  Port=5
  Ref : Inport  Port=6
  Adaptive MPC Controller : mpclib/Adaptive MPC Controller  SCDEnableBlockLinearizationSpecification=on  mpcobj=mpcobj  x0=egoStates  enable_value=0  updateMPCinCallerWorkspace=on  md_inport=off  mv_inport=off  uref_inport=off  return_cost=off  return_mvseq=off  return_qpstatus=off  return_xseq=off  return_state=off  return_ovseq=off  state_inport=off  isltv_plant=off  umin_inport=off  umax_inport=off  ymin_inport=off  ymax_inport=off  cc_inport=on  ywt_inport=on  uwt_inport=on  duwt_inport=on  rhoeps_inport=off  pm_inport=off  MaximumP=10  HorizonChoice=FixedHorizon  BlockDataType=double  SampleTimeInherited=on  switch_inport=off
  Constant : Constant  Value=WOV
  Constant2 : Constant  Value=WMV
  Constant3 : Constant  Value=WMVR
  LastMV : Memory  InitialCondition=u0
  MATLAB Function : MATLAB Function  TreatAsAtomicUnit=on
  Throttle & Delta : Outport  VectorParamsAs1DForOutWhenUnconnected=on
  Curvature : Outport  Port=2
  wires:
  Constraint_E/1 -> Adaptive MPC Controller/4
  Constraint_G/1 -> Adaptive MPC Controller/6
  Constant3/1 -> Adaptive MPC Controller/9
  Constant2/1 -> Adaptive MPC Controller/8
  Constraint_F/1 -> Adaptive MPC Controller/5
  Constant/1 -> Adaptive MPC Controller/7
  State/1 -> Adaptive MPC Controller/2
  Adaptive MPC Controller/1 -> LastMV/1
  LastMV/1 -> Throttle & Delta/1  "Throttle & Delta"
  Plant/1 -> Adaptive MPC Controller/1
  MATLAB Function/1(Curvature) -> Curvature/1
  Ref/1 -> Adaptive MPC Controller/3, MATLAB Function/1(Reference)

== matlab function Dynamic_obstacle_avoidance_PIL/PIL_Model/Calculating deviation from reference/MATLAB Function ==
  settings: updateMethod=DISCRETE  sampleTime=Ts
  data: reference input; dev output; actual input; lateral_dev output
function [dev,lateral_dev] = fcn(reference, actual)

[dev, lateral_dev] = deviation(reference,actual);

== matlab function Dynamic_obstacle_avoidance_PIL/MIL_Model/Calculating deviation from reference/MATLAB Function ==
  settings: updateMethod=DISCRETE  sampleTime=Ts
  data: reference input; dev output; actual input; lateral_dev output
function [dev,lateral_dev] = fcn(reference, actual)

[dev, lateral_dev] = deviation(reference,actual);

== stateflow chart Dynamic_obstacle_avoidance_PIL/PIL_Model/Calculating deviation from reference/Test Assessment1 ==
  settings: stateMachineType=SIMPLIFIED_MACHINE
  state Safe_Overtake_Assessment
    if Zone == 3
    verify(duration(lateral_dev > 5 && lateral_dev < 3,sec)<1);
    end
  (default) -> Safe_Overtake_Assessment
  data: lateral_dev input; Zone input

== matlab function Dynamic_obstacle_avoidance_PIL/PIL_Model/Dynamic Model/Dynamic_Model ==
  data: x input; u input; xdot output; param input; X output; Y output; yaw output; v output
function [xdot,X, Y, yaw, v] = fcn(x,u,param)

[xdot,X, Y, yaw, v] = VehicleModelCT_DYN(x,u,param);

== stateflow chart Dynamic_obstacle_avoidance_PIL/PIL_Model/Dynamic Model/Lateral Acceleration Assessment ==
  settings: stateMachineType=SIMPLIFIED_MACHINE
  state Global_Assessment
    % Check if the lateral acceleration of the vehicle is below 2m/s^2  except for half a second period
    verify(duration(Lateral_acceleration>=2,sec)<=0.5)
  (default) -> Global_Assessment
  data: Lateral_acceleration input

== matlab function Dynamic_obstacle_avoidance_PIL/PIL_Model/Obstacle detector/MATLAB Function1 ==
  settings: updateMethod=DISCRETE  sampleTime=Ts
  data: Actual input; SafeX output; Obstacle input; SafeY output; EndX output; EndY output; EntryPoint output; DetectionPoint output; detection output; map input; Lw input; Ts input; Zone output; indexObs input; indexObs_old output; ObstacleCnt_old output; ObstacleCnt input; ActualIdx input; EndIdx input; EndIdx_old output; EntryIdx input; DetIdx input; SafeIdx input; EntryIdx_old output; DetIdx_old output; SafeIdx_old output; leftLaneFLAG input; leftLaneFLAG_old output
function [SafeX,SafeY,EndX,EndY,EntryPoint,DetectionPoint,detection,Zone,indexObs_old,ObstacleCnt_old,EndIdx_old,EntryIdx_old,DetIdx_old,SafeIdx_old,leftLaneFLAG_old] = fcn(Actual,Obstacle,map,Lw,Ts,indexObs,ObstacleCnt,ActualIdx,EndIdx,EntryIdx,DetIdx,SafeIdx,leftLaneFLAG)

[SafeX,SafeY,EndX,EndY,EntryPoint,detection,Zone,indexObs_old,DetectionPoint,ObstacleCnt_old,EndIdx_old,EntryIdx_old,DetIdx_old,SafeIdx_old,leftLaneFLAG_old] = detectionFun(Actual,Obstacle,map,Lw,Ts,indexObs,ObstacleCnt,ActualIdx,EndIdx,EntryIdx,DetIdx,SafeIdx,leftLaneFLAG);

== stateflow chart Dynamic_obstacle_avoidance_PIL/MIL_Model/Calculating deviation from reference/Test Assessment1 ==
  settings: stateMachineType=SIMPLIFIED_MACHINE
  state Safe_Overtake_Assessment
    if Zone == 3
    verify(duration(lateral_dev > 5 && lateral_dev < 3,sec)<1);
    end
  (default) -> Safe_Overtake_Assessment
  data: lateral_dev input; Zone input

== matlab function Dynamic_obstacle_avoidance_PIL/PIL_Model/Plant generator/Plant Model Generator ==
  settings: updateMethod=DISCRETE  sampleTime=Ts
  data: x input; u input; A output; B output; C output; D output; U output size=[2,1]; Y output size=[4,1]; X output size=[4,1]; DX output size=[4,1]; Ts parameter; param input
function [A,B,C,D,U,Y,X,DX] = fcn(x,u,Ts,param)
[A,B,C,D,U,Y,X,DX] = obstacleVehicleModelDT(Ts,x,u,param);

== matlab function Dynamic_obstacle_avoidance_PIL/PIL_Model/Subsystem/Adaptive MPC Controller/MATLAB Function ==
  data: Reference input; Curvature output
function Curvature = fcn(Reference)

Curvature = curvatureEstimator(Reference);

== matlab function Dynamic_obstacle_avoidance_PIL/MIL_Model/Dynamic Model/Dynamic_Model ==
  data: x input; u input; xdot output; param input; X output; Y output; yaw output; v output
function [xdot,X, Y, yaw, v] = fcn(x,u,param)

[xdot,X, Y, yaw, v] = VehicleModelCT_DYN(x,u,param);

== stateflow chart Dynamic_obstacle_avoidance_PIL/MIL_Model/Dynamic Model/Lateral Acceleration Assessment ==
  settings: stateMachineType=SIMPLIFIED_MACHINE
  state Global_Assessment
    % Check if the lateral acceleration of the vehicle is below 2m/s^2  except for half a second period
    verify(duration(Lateral_acceleration>=2,sec)<=0.5)
  (default) -> Global_Assessment
  data: Lateral_acceleration input

== matlab function Dynamic_obstacle_avoidance_PIL/MIL_Model/Obstacle detector/MATLAB Function1 ==
  settings: updateMethod=DISCRETE  sampleTime=Ts
  data: Actual input; SafeX output; Obstacle input; SafeY output; EndX output; EndY output; EntryPoint output; DetectionPoint output; detection output; map input; Lw input; Ts input; Zone output; indexObs input; indexObs_old output; ObstacleCnt_old output; ObstacleCnt input; ActualIdx input; EndIdx input; EndIdx_old output; EntryIdx input; DetIdx input; SafeIdx input; EntryIdx_old output; DetIdx_old output; SafeIdx_old output; leftLaneFLAG input; leftLaneFLAG_old output
function [SafeX,SafeY,EndX,EndY,EntryPoint,DetectionPoint,detection,Zone,indexObs_old,ObstacleCnt_old,EndIdx_old,EntryIdx_old,DetIdx_old,SafeIdx_old,leftLaneFLAG_old] = fcn(Actual,Obstacle,map,Lw,Ts,indexObs,ObstacleCnt,ActualIdx,EndIdx,EntryIdx,DetIdx,SafeIdx,leftLaneFLAG)

[SafeX,SafeY,EndX,EndY,EntryPoint,detection,Zone,indexObs_old,DetectionPoint,ObstacleCnt_old,EndIdx_old,EntryIdx_old,DetIdx_old,SafeIdx_old,leftLaneFLAG_old] = detectionFun(Actual,Obstacle,map,Lw,Ts,indexObs,ObstacleCnt,ActualIdx,EndIdx,EntryIdx,DetIdx,SafeIdx,leftLaneFLAG);

== matlab function Dynamic_obstacle_avoidance_PIL/MIL_Model/Plant generator/Plant Model Generator ==
  settings: updateMethod=DISCRETE  sampleTime=Ts
  data: x input; u input; A output; B output; C output; D output; U output size=[2,1]; Y output size=[4,1]; X output size=[4,1]; DX output size=[4,1]; Ts parameter; param input
function [A,B,C,D,U,Y,X,DX] = fcn(x,u,Ts,param)
[A,B,C,D,U,Y,X,DX] = obstacleVehicleModelDT(Ts,x,u,param);

== matlab function Dynamic_obstacle_avoidance_PIL/MIL_Model/Subsystem/Adaptive MPC Controller/MATLAB Function ==
  data: Reference input; Curvature output
function Curvature = fcn(Reference)

Curvature = curvatureEstimator(Reference);

== matlab function Dynamic_obstacle_avoidance_PIL/MIL_Model/Subsystem/MATLAB Function ==
  settings: updateMethod=DISCRETE  sampleTime=Ts
  data: Reference input; E output size=[2 2]; Lw input; SafeX input; SafeY input; EndX input; EndY input; EntryPoint input; DetectionPoint input; detection input; F output size=[2 4]; G output size=[2 1]; Zone input; Curvature input
function [E, F, G] = fcn(Reference,Lw,SafeX,SafeY,EndX,EndY,EntryPoint,DetectionPoint,detection,Zone,Curvature)

[E, F, G] = LaneKeepConstraint(Reference,Lw,detection,SafeX,SafeY,EndX,EndY,EntryPoint,Zone,DetectionPoint,Curvature);
